simulink model "PP_vs_LQ_controllers_sim_SwingUp"  (R2019b)
settings: Solver=FixedStepAuto  StartTime=0.0  StopTime=10  FixedStep=1e-2  RelTol=1e-3
undefined symbols (not defined in the file): Klqi_int, Klqi_state, Parameters
settings Model: Creator=Samsung  LastModifiedBy=Samsung

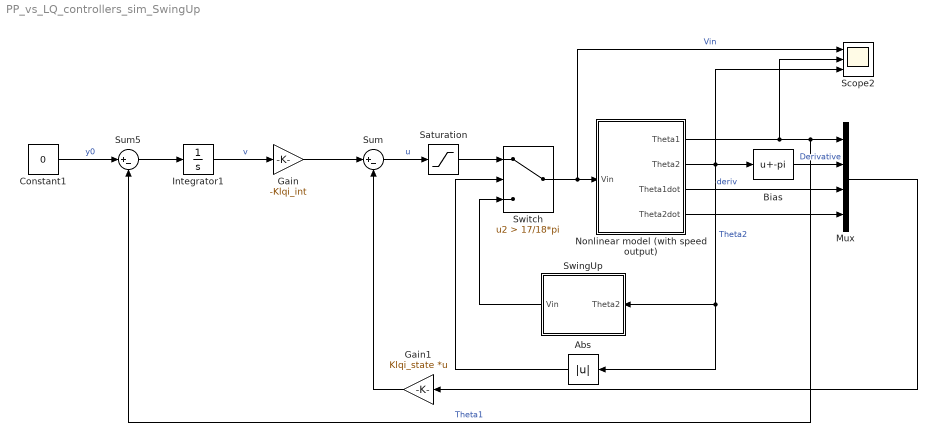
== system PP_vs_LQ_controllers_sim_SwingUp ==
  Abs : Abs
  Bias : Bias  Bias=-pi
  Constant1 : Constant  Value=0
  Gain : Gain  Gain=-Klqi_int
  Gain1 : Gain  Gain=Klqi_state  Multiplication=Matrix(K*u)
  Integrator1 : Integrator
  Mux : Mux
  Nonlinear model (with speed output) : Subsystem
  Saturation : Saturate  UpperLimit=10  LowerLimit=-10
  Scope2 : Scope  NumInputPorts=3
  Sum : Sum  Inputs=|+-
  Sum5 : Sum  Inputs=|+-
  SwingUp : Subsystem
  Switch : Switch  Criteria=u2 > Threshold  Threshold=17/18*pi
  wires:
  Nonlinear model (with speed output)/1(Theta1) -> Scope2/2, Mux/1, Sum5/2  "Theta1"
  Mux/1 -> Gain1/1
  Gain1/1 -> Sum/2
  Sum5/1 -> Integrator1/1
  Sum/1 -> Saturation/1  "u"
  Nonlinear model (with speed output)/3(Theta1dot) -> Mux/3  "deriv"
  Nonlinear model (with speed output)/4(Theta2dot) -> Mux/4
  Integrator1/1 -> Gain/1  "v"
  Gain/1 -> Sum/1
  Bias/1 -> Mux/2  "Derivative"
  Constant1/1 -> Sum5/1  "y0"
  Nonlinear model (with speed output)/2(Theta2) -> Scope2/3, Abs/1, SwingUp/1(Theta2), Bias/1  "Theta2"
  Saturation/1 -> Switch/1
  Switch/1 -> Scope2/1, Nonlinear model (with speed output)/1(Vin)  "Vin"
  SwingUp/1(Vin) -> Switch/3
  Abs/1 -> Switch/2

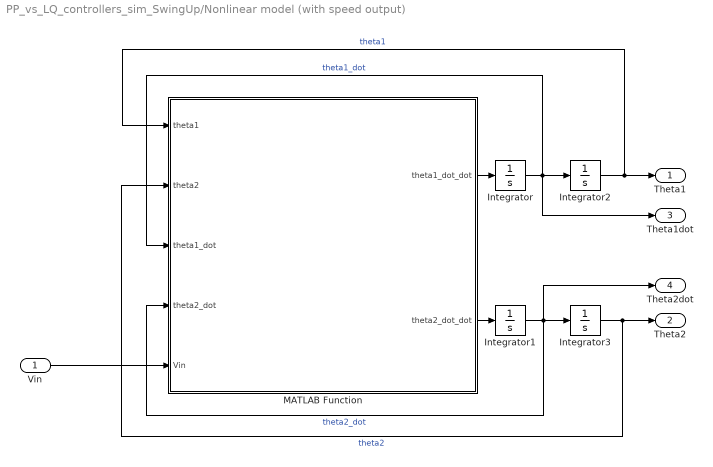
== system PP_vs_LQ_controllers_sim_SwingUp/Nonlinear model (with speed output) ==
  Vin : Inport
  Integrator{,1..3} (4 alike) : Integrator
  MATLAB Function : MATLAB Function  TreatAsAtomicUnit=on  mask{Pars=Parameters}
      mask prompts: Pars "Struct containing model parameters"
  Theta1 : Outport
  Theta2 : Outport  Port=2
  Theta1dot : Outport  Port=3
  Theta2dot : Outport  Port=4
  wires:
  Integrator/1 -> Theta1dot/1, MATLAB Function/3(theta1_dot), Integrator2/1  "theta1_dot"
  Integrator1/1 -> Theta2dot/1, MATLAB Function/4(theta2_dot), Integrator3/1  "theta2_dot"
  MATLAB Function/1(theta1_dot_dot) -> Integrator/1
  Integrator3/1 -> Theta2/1, MATLAB Function/2(theta2)  "theta2"
  MATLAB Function/2(theta2_dot_dot) -> Integrator1/1
  Integrator2/1 -> MATLAB Function/1(theta1), Theta1/1  "theta1"
  Vin/1 -> MATLAB Function/5(Vin)

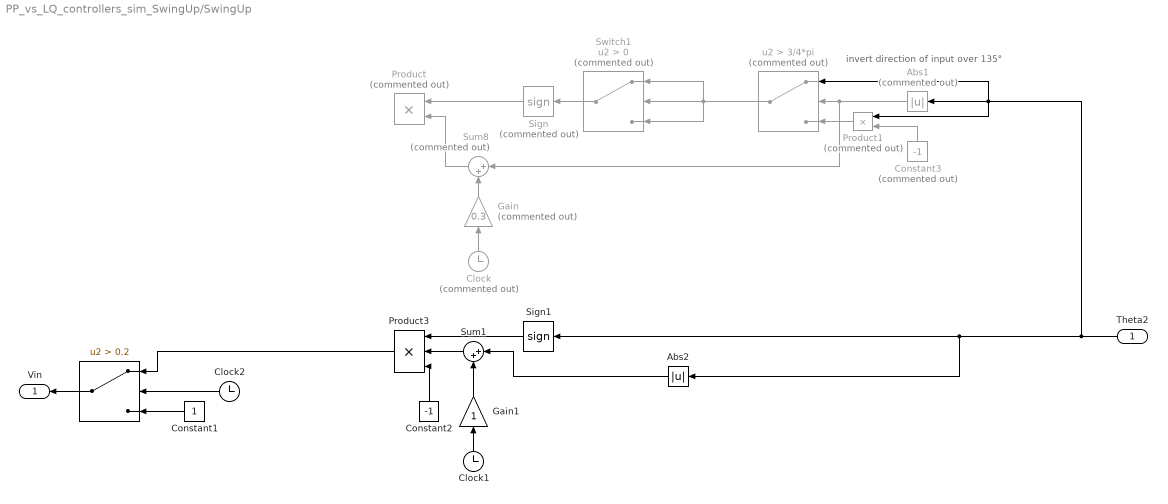
== system PP_vs_LQ_controllers_sim_SwingUp/SwingUp ==
  note: invert direction of input over 135°
  Theta2 : Inport
  " " : Switch  Commented=on  Criteria=u2 > Threshold  Threshold=3/4*pi
  " " : Switch  Criteria=u2 > Threshold  Threshold=0.2
  Abs1 : Abs  Commented=on
  Abs2 : Abs
  Clock : Clock  Commented=on
  Clock1 : Clock
  Clock2 : Clock
  Constant1 : Constant
  Constant2 : Constant  Value=-1
  Constant3 : Constant  Commented=on  Value=-1
  Gain : Gain  Commented=on  Gain=0.3
  Gain1 : Gain
  Product : Product  Commented=on
  Product1 : Product  Commented=on
  Product3 : Product  Inputs=3
  Sign : Signum  Commented=on
  Sign1 : Signum
  Sum1 : Sum  Inputs=|++
  Sum8 : Sum  Commented=on  Inputs=|++
  Switch1 : Switch  Commented=on  Criteria=u2 > Threshold
  Vin : Outport
  wires:
  Abs1/1 -> Sum8/1, " "/2
  " "/1 -> Switch1/3, Switch1/2, Switch1/1
  Constant3/1 -> Product1/2
  Clock/1 -> Gain/1
  Product1/1 -> " "/3
  Switch1/1 -> Sign/1
  Gain/1 -> Sum8/2
  Sign/1 -> Product/1
  Sum8/1 -> Product/2
  Sign1/1 -> Product3/1
  Sum1/1 -> Product3/2
  Clock1/1 -> Gain1/1
  Gain1/1 -> Sum1/2
  Theta2/1 -> Product1/1, Abs1/1, " "/1, Abs2/1, Sign1/1
  Abs2/1 -> Sum1/1
  Constant2/1 -> Product3/3
  Clock2/1 -> " "/2
  Constant1/1 -> " "/3
  " "/1 -> Vin/1
  Product3/1 -> " "/1

== matlab function PP_vs_LQ_controllers_sim_SwingUp/Nonlinear model (with speed output)/MATLAB Function ==
  data: theta1 input; theta1_dot_dot output; theta2 input; theta1_dot input; theta2_dot input; Vin input; theta2_dot_dot output; Pars parameter
function [theta1_dot_dot,theta2_dot_dot] = fcn(theta1, theta2, theta1_dot, theta2_dot,Vin, Pars)

   k1 = Pars.Jeq + Pars.m2*(Pars.l1^2 + Pars.x2^2*sin(theta2)^2);
   k2 = Pars.m2*Pars.l1*Pars.x2*cos(theta2);
   k3 = 2*Pars.m2*Pars.x2^2*sin(theta2)*cos(theta2)*theta1_dot*theta2_dot - Pars.m2*Pars.l1*Pars.x2*sin(theta2)*theta2_dot^2 +Pars.Ks*theta1 - Pars.Km/Pars.Rm*Vin + (Pars.Km^2)/Pars.Rm*theta1_dot + Pars.Kf1*theta1_dot;
   k4 = Pars.m2*Pars.l1*Pars.x2*cos(theta2);
   k5 = Pars.m2*Pars.x2^2 + Pars.I2;
   k6 = - Pars.m2*Pars.x2^2*sin(theta2)*cos(theta2)*theta1_dot^2 + Pars.m2*Pars.g*Pars.x2*sin(theta2) + Pars.Kf2*theta2_dot;


theta1_dot_dot = (k2*k6 - k3*k5)/(k1*k5 - k2*k4);
theta2_dot_dot = -(k1*k6 - k3*k4)/(k1*k5 - k2*k4);
